simulink model "phase2_Q5"  (R2022b)
settings: Solver=ode4  StartTime=0.0  StopTime=15  FixedStep=0.01  RelTol=1e-3
InitFcn:
  | initial
values from neighbouring files (symbols this model uses):
  g = 9.81    [initial.m]
undefined symbols (not defined in the file or in its folder): body, chi0, lambda0, omega0, RRV, v0
libraries: matrix_library x2, sharedtransform x1
settings Model: Creator=User  LastModifiedBy=Alire

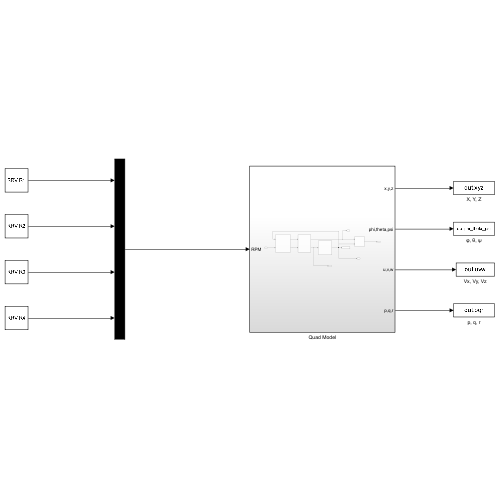
[thumbnail: Simulink's stored preview of the top-level diagram]
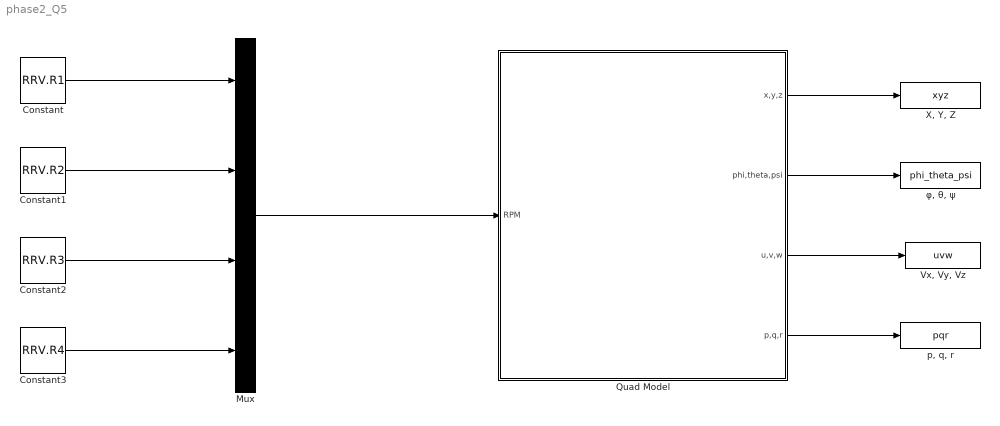
== system phase2_Q5 ==
  Constant : Constant  Value=RRV.R1
  Constant1 : Constant  Value=RRV.R2
  Constant2 : Constant  Value=RRV.R3
  Constant3 : Constant  Value=RRV.R4
  Mux : Mux
  Quad Model : Subsystem
  "Vx, Vy, Vz" : ToWorkspace  VariableName=uvw  SampleTime=-1
  "X, Y, Z" : ToWorkspace  VariableName=xyz  SampleTime=-1
  "p, q, r" : ToWorkspace  VariableName=pqr  SampleTime=-1
  "φ, θ, ψ" : ToWorkspace  VariableName=phi_theta_psi  SampleTime=-1
  wires:
  Constant1/1 -> Mux/2
  Constant3/1 -> Mux/4
  Constant/1 -> Mux/1
  Constant2/1 -> Mux/3
  Quad Model/1(x,y,z) -> "X, Y, Z"/1
  Mux/1 -> Quad Model/1(RPM)
  Quad Model/3(u,v,w) -> "Vx, Vy, Vz"/1
  Quad Model/4(p,q,r) -> "p, q, r"/1
  Quad Model/2(phi,theta,psi) -> "φ, θ, ψ"/1

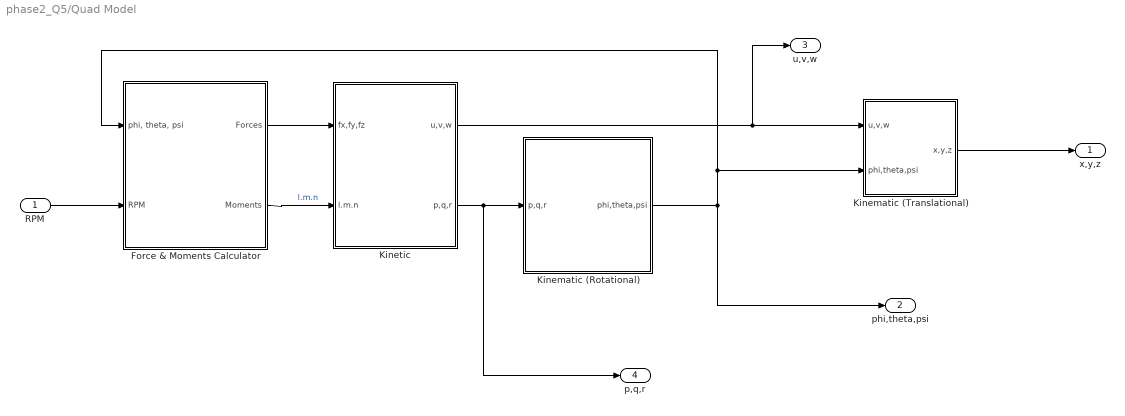
== system phase2_Q5/Quad Model ==
  RPM : Inport
  Force & Moments Calculator : Subsystem
  Kinematic (Rotational) : Subsystem
  Kinematic (Translational) : Subsystem
  Kinetic : Subsystem
  x,y,z : Outport
  phi,theta,psi : Outport  Port=2
  u,v,w : Outport  Port=3
  p,q,r : Outport  Port=4
  wires:
  Force & Moments Calculator/1(Forces) -> Kinetic/1(fx,fy,fz)
  Kinematic (Rotational)/1(phi,theta,psi) -> phi,theta,psi/1, Force & Moments Calculator/1("phi, theta, psi"), Kinematic (Translational)/2(phi,theta,psi)
  Kinematic (Translational)/1(x,y,z) -> x,y,z/1
  Kinetic/2(p,q,r) -> p,q,r/1, Kinematic (Rotational)/1(p,q,r)
  RPM/1 -> Force & Moments Calculator/2(RPM)
  Kinetic/1(u,v,w) -> u,v,w/1, Kinematic (Translational)/1(u,v,w)
  Force & Moments Calculator/2(Moments) -> Kinetic/2(l.m.n)  "l.m.n"

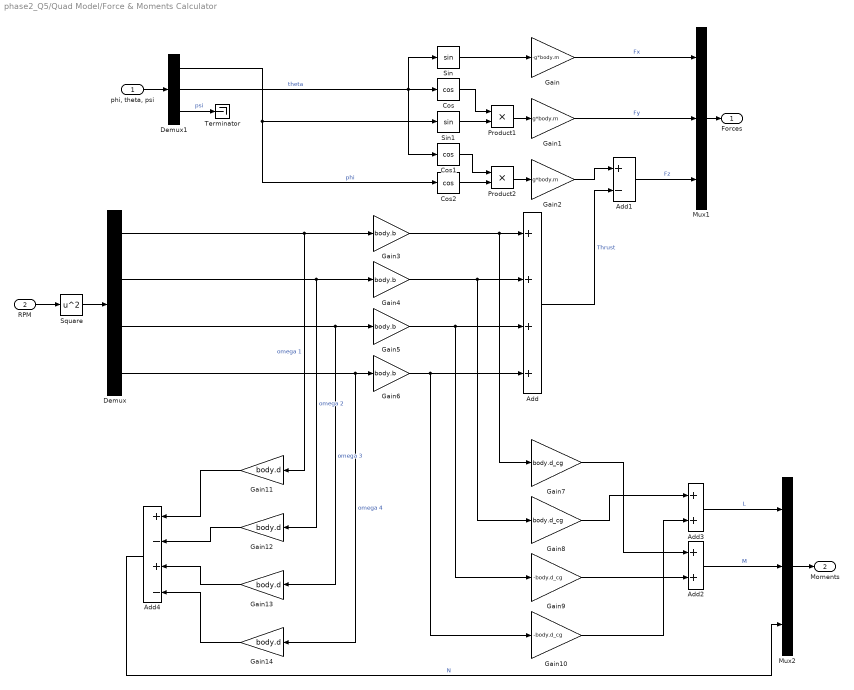
== system phase2_Q5/Quad Model/Force & Moments Calculator ==
  "phi, theta, psi" : Inport
  RPM : Inport  Port=2
  Add : Sum  Inputs=++++
  Add1 : Sum  Inputs=+-
  Add2 : Sum
  Add3 : Sum
  Add4 : Sum  Inputs=+-+-
  Cos : Trigonometry  Operator=cos
  Cos1 : Trigonometry  Operator=cos
  Cos2 : Trigonometry  Operator=cos
  Demux : Demux
  Demux1 : Demux  Outputs=3
  Gain : Gain  Gain=-g*body.m
  Gain1 : Gain  Gain=g*body.m
  Gain10 : Gain  Gain=-body.d_cg
  Gain{11..14} (4 alike) : Gain  Gain=body.d
  Gain2 : Gain  Gain=g*body.m
  Gain{3..6} (4 alike) : Gain  Gain=body.b
  Gain7 : Gain  Gain=body.d_cg
  Gain8 : Gain  Gain=body.d_cg
  Gain9 : Gain  Gain=-body.d_cg
  Mux1 : Mux  Inputs=3
  Mux2 : Mux  Inputs=3
  Product1 : Product
  Product2 : Product
  Sin : Trigonometry
  Sin1 : Trigonometry
  Square : Math  Operator=square
  Terminator : Terminator
  Forces : Outport
  Moments : Outport  Port=2
  wires:
  Cos2/1 -> Product2/2
  Cos1/1 -> Product2/1
  Gain1/1 -> Mux1/2  "Fy"
  Demux/3 -> Gain13/1, Gain5/1  "omega 3"
  Gain5/1 -> Gain9/1, Add/3
  Gain2/1 -> Add1/1
  Demux1/1 -> Sin1/1, Cos2/1  "phi"
  Add3/1 -> Mux2/1  "L"
  Gain4/1 -> Gain8/1, Add/2
  Gain6/1 -> Gain10/1, Add/4
  Gain3/1 -> Gain7/1, Add/1
  Demux/2 -> Gain4/1, Gain12/1  "omega 2"
  Gain9/1 -> Add2/2
  Sin1/1 -> Product1/2
  Gain/1 -> Mux1/1  "Fx"
  Add2/1 -> Mux2/2  "M"
  Gain13/1 -> Add4/3
  Demux/1 -> Gain3/1, Gain11/1  "omega 1"
  Demux1/2 -> Sin/1, Cos1/1, Cos/1  "theta"
  Gain7/1 -> Add2/1
  Gain14/1 -> Add4/4
  Demux/4 -> Gain14/1, Gain6/1  "omega 4"
  Cos/1 -> Product1/1
  Gain12/1 -> Add4/2
  Add/1 -> Add1/2  "Thrust"
  Add4/1 -> Mux2/3  "N"
  Mux2/1 -> Moments/1
  Gain11/1 -> Add4/1
  Sin/1 -> Gain/1
  Product1/1 -> Gain1/1
  Add1/1 -> Mux1/3  "Fz"
  Gain8/1 -> Add3/1
  RPM/1 -> Square/1
  Gain10/1 -> Add3/2
  Product2/1 -> Gain2/1
  Mux1/1 -> Forces/1
  "phi, theta, psi"/1 -> Demux1/1
  Demux1/3 -> Terminator/1  "psi"
  Square/1 -> Demux/1

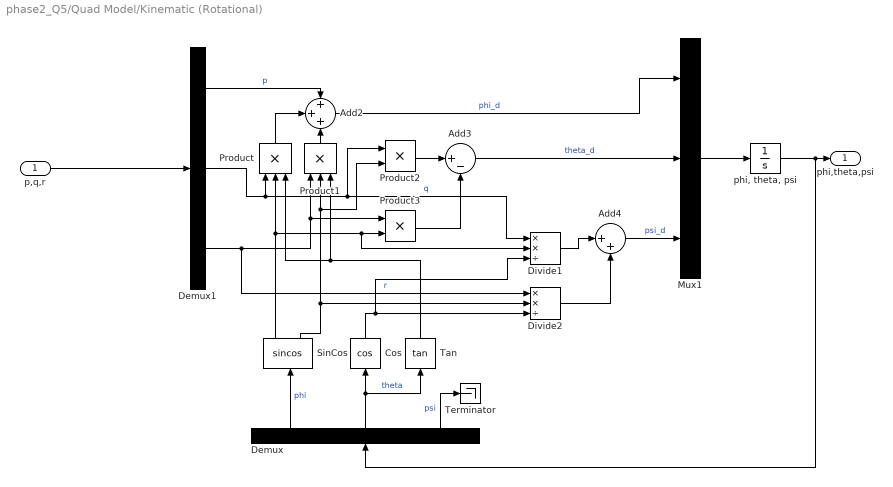
== system phase2_Q5/Quad Model/Kinematic (Rotational) ==
  p,q,r : Inport
  Add2 : Sum  Inputs=+++
  Add3 : Sum  Inputs=|+-
  Add4 : Sum  Inputs=|++
  Cos : Trigonometry  Operator=cos
  Demux : Demux  Outputs=3
  Demux1 : Demux  Outputs=3
  Divide1 : Product  Inputs=**/
  Divide2 : Product  Inputs=**/
  Mux1 : Mux  Inputs=3
  Product : Product  Inputs=3
  Product1 : Product  Inputs=3
  Product2 : Product
  Product3 : Product
  SinCos : Trigonometry  Operator=sincos
  Tan : Trigonometry  Operator=tan
  Terminator : Terminator
  "phi, theta, psi" : Integrator  InitialCondition=[lambda0.phi, lambda0.theta, lambda0.psi]
  phi,theta,psi : Outport
  wires:
  SinCos/2 -> Divide2/2, Product2/2, Product1/2
  Divide1/1 -> Add4/1
  Product1/1 -> Add2/3
  Demux1/2 -> Product/1, Divide1/1, Product2/1  "q"
  Demux1/3 -> Divide2/1, Product3/1, Product1/1  "r"
  Product2/1 -> Add3/1
  Tan/1 -> Product1/3, Product/3
  Demux/3 -> Terminator/1  "psi"
  Mux1/1 -> "phi, theta, psi"/1
  Cos/1 -> Divide2/3, Divide1/3
  Demux/1 -> SinCos/1  "phi"
  SinCos/1 -> Divide1/2, Product3/2, Product/2
  Add2/1 -> Mux1/1  "phi_d"
  Demux1/1 -> Add2/1  "p"
  Product/1 -> Add2/2
  Demux/2 -> Cos/1, Tan/1  "theta"
  Product3/1 -> Add3/2
  Add3/1 -> Mux1/2  "theta_d"
  Add4/1 -> Mux1/3  "psi_d"
  Divide2/1 -> Add4/2
  "phi, theta, psi"/1 -> Demux/1, phi,theta,psi/1
  p,q,r/1 -> Demux1/1

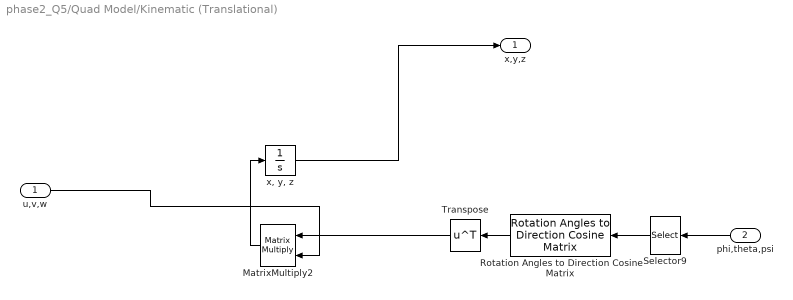
== system phase2_Q5/Quad Model/Kinematic (Translational) ==
  u,v,w : Inport
  phi,theta,psi : Inport  Port=2
  MatrixMultiply2 : Product  Multiplication=Matrix(*)
  Rotation Angles to Direction Cosine Matrix : sharedtransform/Rotation Angles to Direction Cosine Matrix  rotationOrder=ZYX  aMode=aMode
  Selector9 : Selector  InputPortWidth=3  IndexOptions=Index vector (dialog)  Indices=[3 2 1]  OutputSizes=1
  Transpose : Math  Operator=transpose
  "x, y, z" : Integrator  InitialCondition=[chi0.x, chi0.y, chi0.z]
  x,y,z : Outport
  wires:
  Transpose/1 -> MatrixMultiply2/1
  Selector9/1 -> Rotation Angles to Direction Cosine Matrix/1
  MatrixMultiply2/1 -> "x, y, z"/1
  u,v,w/1 -> MatrixMultiply2/2
  Rotation Angles to Direction Cosine Matrix/1 -> Transpose/1
  "x, y, z"/1 -> x,y,z/1
  phi,theta,psi/1 -> Selector9/1

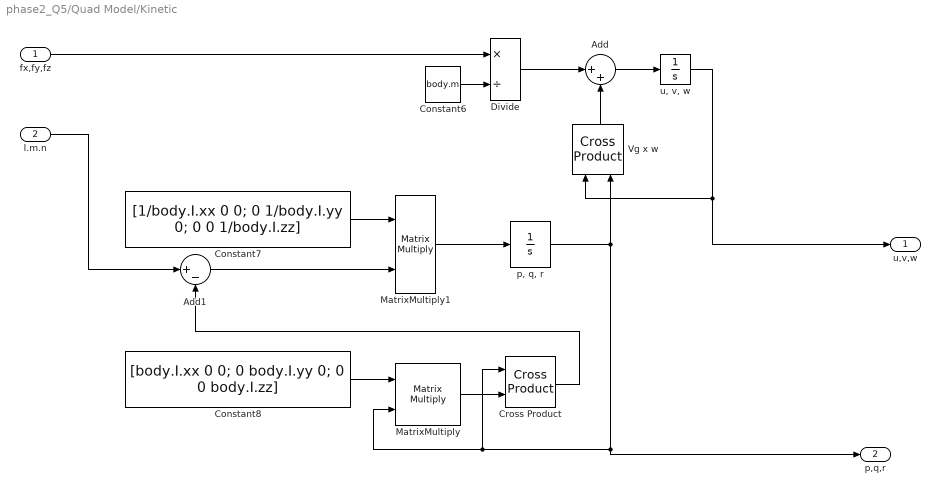
== system phase2_Q5/Quad Model/Kinetic ==
  fx,fy,fz : Inport
  l.m.n : Inport  Port=2
  Add : Sum  Inputs=|++
  Add1 : Sum  Inputs=|+-
  Constant6 : Constant  Value=body.m
  Constant7 : Constant  Value="[1/body.I.xx 0 0; 0 1/body.I.yy 0; 0 0  1/body.I.zz]"
  Constant8 : Constant  Value="[body.I.xx 0 0; 0 body.I.yy 0; 0 0  body.I.zz]"
  Cross Product : matrix_library/Cross Product
  Divide : Product  Inputs=*/
  MatrixMultiply : Product  Multiplication=Matrix(*)
  MatrixMultiply1 : Product  Multiplication=Matrix(*)
  Vg x w : matrix_library/Cross Product
  "p, q, r" : Integrator  InitialCondition=[omega0.p, omega0.q, omega0.r]
  "u, v, w" : Integrator  InitialCondition=[v0.x, v0.y, v0.z]
  u,v,w : Outport
  p,q,r : Outport  Port=2
  wires:
  "u, v, w"/1 -> u,v,w/1, Vg x w/1
  Vg x w/1 -> Add/2
  Constant6/1 -> Divide/2
  Add1/1 -> MatrixMultiply1/2
  "p, q, r"/1 -> p,q,r/1, Cross Product/1, MatrixMultiply/2, Vg x w/2
  Divide/1 -> Add/1
  Constant8/1 -> MatrixMultiply/1
  Add/1 -> "u, v, w"/1
  Cross Product/1 -> Add1/2
  MatrixMultiply/1 -> Cross Product/2
  Constant7/1 -> MatrixMultiply1/1
  fx,fy,fz/1 -> Divide/1
  MatrixMultiply1/1 -> "p, q, r"/1
  l.m.n/1 -> Add1/1
